simulink model "Q3_b3"  (R2017b)
settings: Solver=VariableStepAuto  StartTime=0.0  StopTime=0.1  RelTol=1e-8  AbsTol=1e-8
undefined symbols (not defined in the file or in its folder): K2
libraries: cstblocks x14
settings Model: Creator=User  LastModifiedBy=User

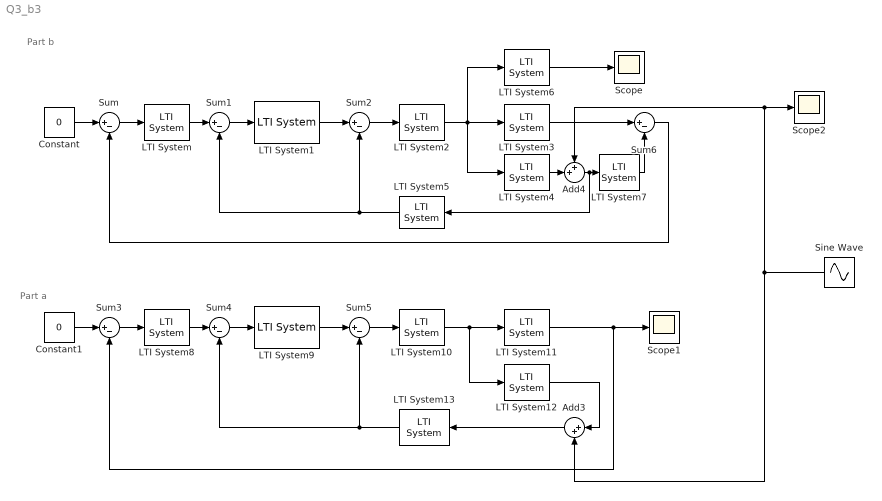
== system Q3_b3 ==
  note: Part b
  note: Part a
  Add3 : Sum  Inputs=|++
  Add4 : Sum  Inputs=++|
  Constant : Constant  Value=0
  Constant1 : Constant  Value=0
  LTI System : cstblocks/LTI System  sys=K3  IC=[]
  LTI System1 : cstblocks/LTI System  sys=K2*tf(1,[1 0])  IC=[]
  LTI System10 : cstblocks/LTI System  sys=K1  IC=[]
  LTI System11 : cstblocks/LTI System  sys=Pa  IC=[]
  LTI System12 : cstblocks/LTI System  sys=Pq  IC=[]
  LTI System13 : cstblocks/LTI System  sys=H  IC=[]
  LTI System2 : cstblocks/LTI System  sys=K1  IC=[]
  LTI System3 : cstblocks/LTI System  sys=Pa_m  IC=[]
  LTI System4 : cstblocks/LTI System  sys=Pq  IC=[]
  LTI System5 : cstblocks/LTI System  sys=H  IC=[]
  LTI System6 : cstblocks/LTI System  sys=Pa  IC=[]
  LTI System7 : cstblocks/LTI System  sys=F  IC=[]
  LTI System8 : cstblocks/LTI System  sys=K3  IC=[]
  LTI System9 : cstblocks/LTI System  sys=K2*tf(1,[1 0])  IC=[]
  Scope : Scope
  Scope1 : Scope
  Scope2 : Scope
  Sine Wave : Sin  Amplitude=0.01  Frequency=1000  SampleTime=0
  Sum{,1..6} (7 alike) : Sum  Inputs=|+-
  wires:
  Sum3/1 -> LTI System8/1
  LTI System13/1 -> Sum4/2, Sum5/2
  LTI System9/1 -> Sum5/1
  Constant1/1 -> Sum3/1
  LTI System8/1 -> Sum4/1
  Sum4/1 -> LTI System9/1
  Sum5/1 -> LTI System10/1
  LTI System10/1 -> LTI System11/1, LTI System12/1
  Sine Wave/1 -> Add3/2, Add4/1, Scope2/1
  LTI System11/1 -> Scope1/1, Sum3/2
  LTI System1/1 -> Sum2/1
  LTI System2/1 -> LTI System6/1, LTI System3/1, LTI System4/1
  LTI System6/1 -> Scope/1
  Sum2/1 -> LTI System2/1
  LTI System5/1 -> Sum1/2, Sum2/2
  Sum/1 -> LTI System/1
  Sum6/1 -> Sum/2
  LTI System7/1 -> Sum6/2
  LTI System/1 -> Sum1/1
  Sum1/1 -> LTI System1/1
  Constant/1 -> Sum/1
  LTI System3/1 -> Sum6/1
  LTI System12/1 -> Add3/1
  Add3/1 -> LTI System13/1
  LTI System4/1 -> Add4/2
  Add4/1 -> LTI System5/1, LTI System7/1
